simulink library "rotationSequence_ul"  (R2018b)
settings: Solver=VariableStepAuto  StartTime=0.0  StopTime=10.0  RelTol=1e-3
settings Model: Creator=jldanie5  LastModifiedBy=jldanie5

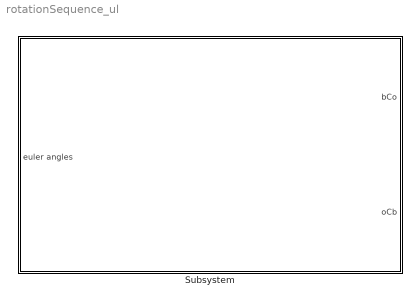
== system rotationSequence_ul ==
  Subsystem : Subsystem

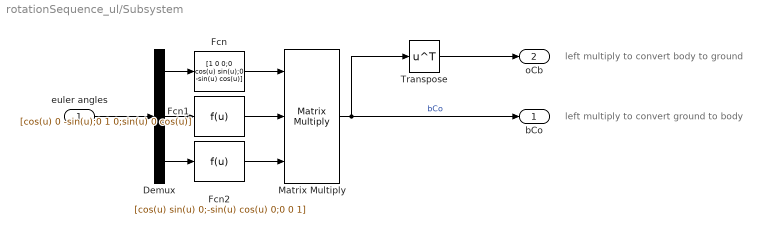
== system rotationSequence_ul/Subsystem ==
  note: left multiply to convert body to ground
  note: left multiply to convert ground to body
  "euler angles " : Inport
  Demux : Demux  Outputs=3
  Fcn : Fcn  Expr=[1 0 0;0 cos(u) sin(u);0 -sin(u) cos(u)]
  Fcn1 : Fcn  Expr=[cos(u) 0 -sin(u);0 1 0;sin(u) 0 cos(u)]
  Fcn2 : Fcn  Expr=[cos(u) sin(u) 0;-sin(u) cos(u) 0;0 0 1]
  Matrix Multiply : Product  Inputs=3  Multiplication=Matrix(*)
  Transpose : Math  Operator=transpose  SaturateOnIntegerOverflow=on
  bCo : Outport
  oCb : Outport  Port=2
  wires:
  "euler angles "/1 -> Demux/1
  Demux/2 -> Fcn1/1
  Demux/1 -> Fcn/1
  Demux/3 -> Fcn2/1
  Fcn2/1 -> Matrix Multiply/3
  Fcn1/1 -> Matrix Multiply/2
  Fcn/1 -> Matrix Multiply/1
  Matrix Multiply/1 -> bCo/1, Transpose/1  "bCo"
  Transpose/1 -> oCb/1
